simulink model "system10"  (R2019a)
settings: Solver=ode45  StartTime=0.0  StopTime=stop_time  FixedStep=0.00001  RelTol=1e-9
values from neighbouring files (symbols this model uses):
  beta = 0.001    [Lab3_final.m]
  d_teta0 = 0    [Lab3_final.m]
  g = 9.8    [Lab3_final.m]
  J = m*l^2+(M*L^2)/3    (= 0.00309133333333)    [Lab3_final.m]
  k = 0.35    [Lab3_final.m]
  l = 0.12    [Lab3_final.m]
  L = 0.25    [Lab3_final.m]
  m = 0.07    [Lab3_final.m]
  M = 0.1    [Lab3_final.m]
  T = 0.5    [Lab3_final.m]
  teta0 = pi/4    (= 0.785398163397)    [Lab3_final.m]
settings Model: Creator=Vasco  LastModifiedBy=Vasco

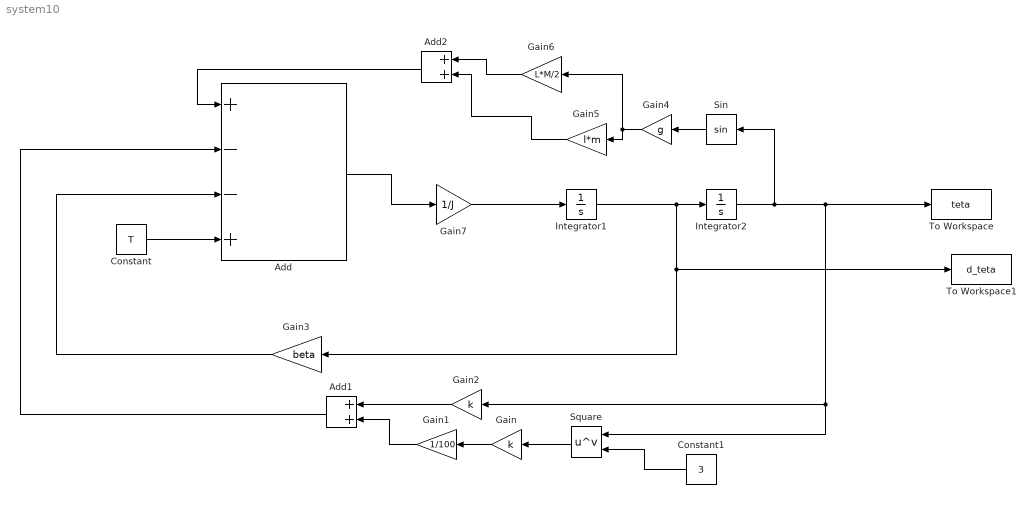
== system system10 ==
  Add : Sum  Inputs=+--+
  Add1 : Sum
  Add2 : Sum
  Constant : Constant  Value=T
  Constant1 : Constant  Value=3
  Gain : Gain  Gain=k
  Gain1 : Gain  Gain=1/100
  Gain2 : Gain  Gain=k
  Gain3 : Gain  Gain=beta
  Gain4 : Gain  Gain=g
  Gain5 : Gain  Gain=l*m
  Gain6 : Gain  Gain=L*M/2
  Gain7 : Gain  Gain=1/J
  Integrator1 : Integrator  InitialCondition=d_teta0
  Integrator2 : Integrator  InitialCondition=teta0
  Sin : Trigonometry
  Square : Math  Operator=pow  SaturateOnIntegerOverflow=on
  To Workspace : ToWorkspace  VariableName=teta  SampleTime=-1
      settings: Save2DSignal=2-D array (concatenate along first dimension)
  To Workspace1 : ToWorkspace  VariableName=d_teta  SampleTime=-1
      settings: Save2DSignal=2-D array (concatenate along first dimension)
  wires:
  Gain7/1 -> Integrator1/1
  Integrator1/1 -> Gain3/1, To Workspace1/1, Integrator2/1
  Integrator2/1 -> Sin/1, To Workspace/1, Square/1, Gain2/1
  Square/1 -> Gain/1
  Constant1/1 -> Square/2
  Gain/1 -> Gain1/1
  Gain1/1 -> Add1/2
  Gain2/1 -> Add1/1
  Add1/1 -> Add/2
  Gain3/1 -> Add/3
  Constant/1 -> Add/4
  Sin/1 -> Gain4/1
  Gain4/1 -> Gain6/1, Gain5/1
  Gain5/1 -> Add2/2
  Gain6/1 -> Add2/1
  Add2/1 -> Add/1
  Add/1 -> Gain7/1
